simulink model "sintonizar2d6"  (Simulink 2.09)
settings: Solver=ode45  StartTime=0.0  StopTime=0.5  MaxStep=0.1  RelTol=1e-3  AbsTol=1e-3
settings Model: SaveTime=off  SaveOutput=off  ConsistencyChecking=off  RTWTemplateMakefile=grt_vc.tmf

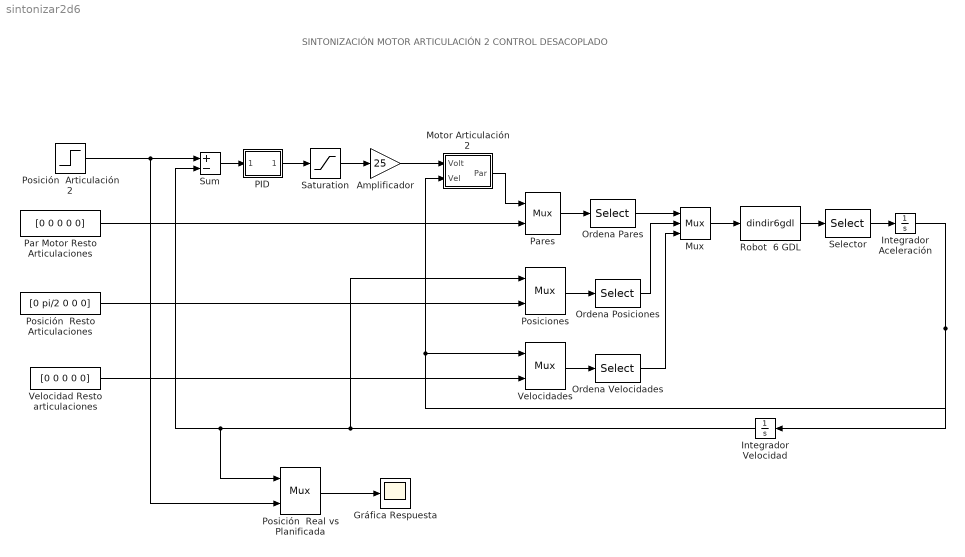
== system sintonizar2d6 ==
  note: SINTONIZACIÓN MOTOR ARTICULACIÓN 2
      | CONTROL DESACOPLADO
  Amplificador : Gain  Gain=25
  Gráfica Respuesta : Scope
      settings: TickLabels=on  TimeRange=auto  YMin=-0.08  YMax=0.005  SaveToWorkspace=off  SaveName=ScopeData  LimitMaxRows=off  MaxRows=500
  Integrador Aceleración : Integrator  ExternalReset=none  InitialConditionSource=internal  InitialCondition=0  LimitOutput=off  UpperSaturationLimit=inf  LowerSaturationLimit=-inf  ShowSaturationPort=off  ShowStatePort=off  AbsoluteTolerance=auto
  Integrador Velocidad : Integrator  Orientation=left  ExternalReset=none  InitialConditionSource=internal  InitialCondition=0  LimitOutput=off  UpperSaturationLimit=inf  LowerSaturationLimit=-inf  ShowSaturationPort=off  ShowStatePort=off  AbsoluteTolerance=auto
  Motor Articulación 2 : Subsystem  mask(Motor){R=0.7, L=0.00101, Kt=0.112, Kv=0.112, imax=21.8, red=500}
      mask prompts: R "Resistencia (Ohmios)"; L "Inductancia (Henrios)"; Kt "Kt (Nm/A)"; Kv "Kv (V/rad/s)"; imax "Corriente máxima (Amperios)"; red "Reductor"
  Mux : Mux  Inputs=3
  Ordena Pares : Selector  Elements=[2 1 3 4 5 6]  InputPortWidth=6
  Ordena Posiciones : Selector  Elements=[2 1 3 4 5 6]  InputPortWidth=6
  Ordena Velocidades : Selector  Elements=[2 1 3 4 5 6]  InputPortWidth=6
  PID : Subsystem  mask(PID Controller){P=200, I=0, D=0}
      mask prompts: P "Proportional:"; I "Integral"; D "Derivative:"
      mask help:
      | Enter expressions for proportional, integral, and derivative terms.
      | P+I/s+Ds
      mask Help: This block implements a PID controller where parameters are entered for the Proportional, Integral and Derivative terms. Unmask this block to see how it works. The derivative term is implemented using a true derivative block.
      mask Display: disp('PID')
  Par Motor Resto Articulaciones : Constant  Value=[0 0 0 0 0]
  Pares : Mux  Inputs=2
  Posiciones : Mux  Inputs=2
  Posición  Articulación 2 : Step  Time=0  Before=0  After=-0.08
  Posición  Real vs Planificada : Mux  Inputs=2
  Posición  Resto Articulaciones : Constant  Value=[0 pi/2 0 0 0]
  Robot  6 GDL : MATLABFcn  MATLABFcn=dindir6gdl  OutputWidth=6
  Saturation : Saturate  UpperLimit=10  LowerLimit=-10
  Selector : Selector  Elements=2  InputPortWidth=6
  Sum : Sum  Inputs=+-
  Velocidad Resto articulaciones : Constant  Value=[0 0 0 0 0]
  Velocidades : Mux  Inputs=2
  wires:
  Ordena Velocidades/1 -> Mux/3
  Velocidades/1 -> Ordena Velocidades/1
  Ordena Posiciones/1 -> Mux/2
  Posiciones/1 -> Ordena Posiciones/1
  Ordena Pares/1 -> Mux/1
  Pares/1 -> Ordena Pares/1
  Integrador Aceleración/1 -> Velocidades/1, Motor Articulación 2/2(Vel), Integrador Velocidad/1
  Selector/1 -> Integrador Aceleración/1
  Posición  Real vs Planificada/1 -> Gráfica Respuesta/1
  Robot  6 GDL/1 -> Selector/1
  Posición  Articulación 2/1 -> Posición  Real vs Planificada/2, Sum/1
  Velocidad Resto articulaciones/1 -> Velocidades/2
  Integrador Velocidad/1 -> Posición  Real vs Planificada/1, Sum/2, Posiciones/1
  Posición  Resto Articulaciones/1 -> Posiciones/2
  Motor Articulación 2/1(Par) -> Pares/1
  Amplificador/1 -> Motor Articulación 2/1(Volt)
  Mux/1 -> Robot  6 GDL/1
  Sum/1 -> PID/1(In_1)
  PID/1(Out_1) -> Saturation/1
  Saturation/1 -> Amplificador/1
  Par Motor Resto Articulaciones/1 -> Pares/2

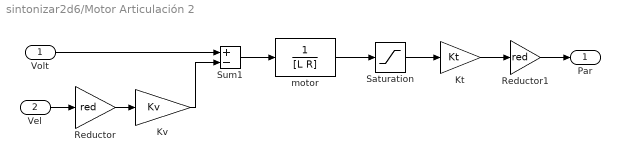
== system sintonizar2d6/Motor Articulación 2 ==
  Volt : Inport  Port=1  PortWidth=-1  SampleTime=-1
  Vel : Inport  Port=2  PortWidth=-1  SampleTime=-1
  Kt : Gain  Gain=Kt
  Kv : Gain  Gain=Kv
  Reductor : Gain  Gain=red
  Reductor1 : Gain  Gain=red
  Saturation : Saturate  UpperLimit=imax  LowerLimit=-imax
  Sum1 : Sum  Inputs=+-
  motor : TransferFcn  Numerator=[1]  Denominator=[L R]
  Par : Outport  Port=1  InitialOutput=0
  wires:
  Saturation/1 -> Kt/1
  motor/1 -> Saturation/1
  Kt/1 -> Reductor1/1
  Reductor1/1 -> Par/1
  Sum1/1 -> motor/1
  Reductor/1 -> Kv/1
  Kv/1 -> Sum1/2
  Volt/1 -> Sum1/1
  Vel/1 -> Reductor/1

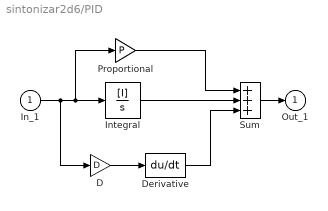
== system sintonizar2d6/PID ==
  In_1 : Inport  Port=1  PortWidth=-1  SampleTime=-1
  D : Gain  Gain=D
  Derivative : Derivative
  Integral : TransferFcn  Numerator=[I]  Denominator=[1 0]
  Proportional : Gain  Gain=P
  Sum : Sum  Inputs=+++
  Out_1 : Outport  Port=1  InitialOutput=0
  wires:
  Proportional/1 -> Sum/1
  Integral/1 -> Sum/2
  Derivative/1 -> Sum/3
  In_1/1 -> Proportional/1, Integral/1, D/1
  Sum/1 -> Out_1/1
  D/1 -> Derivative/1
